simulink model "transform_test"  (R2021b)
settings: Solver=VariableStepAuto  StartTime=0.0  StopTime=60  RelTol=1e-3
libraries: simulink x1
settings Model: Creator=brian  LastModifiedBy=brian

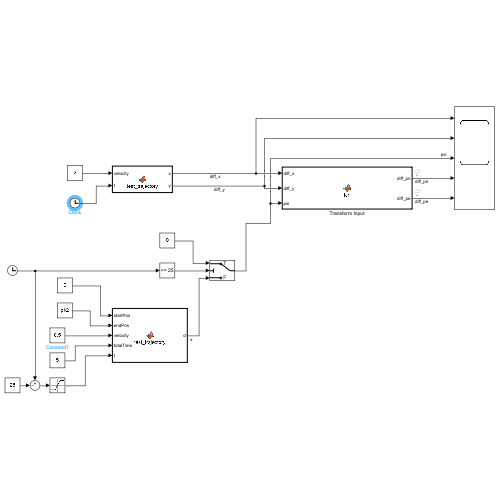
[thumbnail: Simulink's stored preview of the top-level diagram]
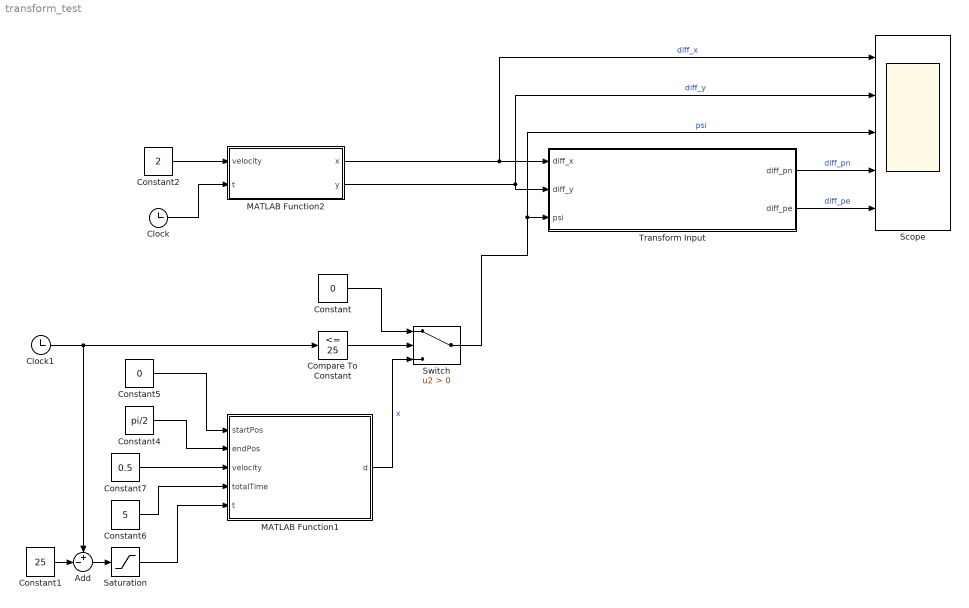
== system transform_test ==
  Add : Sum  Inputs=+-|
  Clock : Clock
  Clock1 : Clock
  Compare To Constant : simulink/Logic and Bit Operations/Compare To Constant  relop=<=  const=25  OutDataTypeStr=boolean
  Constant : Constant  Value=0
  Constant1 : Constant  Value=25
  Constant2 : Constant  Value=2
  Constant4 : Constant  Value=pi/2
  Constant5 : Constant  Value=0
  Constant6 : Constant  Value=5
  Constant7 : Constant  Value=0.5
  MATLAB Function1 : MATLAB Function  TreatAsAtomicUnit=on  SystemSampleTime=0.001
  MATLAB Function2 : MATLAB Function  TreatAsAtomicUnit=on  SystemSampleTime=0.001
  Saturation : Saturate  UpperLimit=250  LowerLimit=0
  Scope : Scope  NumInputPorts=5
  Switch : Switch  Criteria=u2 > Threshold
  Transform Input : MATLAB Function  TreatAsAtomicUnit=on
  wires:
  Transform Input/2(diff_pe) -> Scope/5  "diff_pe"
  Transform Input/1(diff_pn) -> Scope/4  "diff_pn"
  MATLAB Function2/2(y) -> Transform Input/2(diff_y), Scope/2  "diff_y"
  MATLAB Function2/1(x) -> Scope/1, Transform Input/1(diff_x)  "diff_x"
  Switch/1 -> Scope/3, Transform Input/3(psi)  "psi"
  Constant2/1 -> MATLAB Function2/1(velocity)
  Clock/1 -> MATLAB Function2/2(t)
  Constant1/1 -> Add/2
  Compare To Constant/1 -> Switch/2
  Saturation/1 -> MATLAB Function1/5(t)
  Add/1 -> Saturation/1
  Constant5/1 -> MATLAB Function1/1(startPos)
  Constant7/1 -> MATLAB Function1/3(velocity)
  MATLAB Function1/1(d) -> Switch/3  "x"
  Constant6/1 -> MATLAB Function1/4(totalTime)
  Constant/1 -> Switch/1
  Constant4/1 -> MATLAB Function1/2(endPos)
  Clock1/1 -> Compare To Constant/1, Add/1

== matlab function transform_test/MATLAB Function2 ==
  settings: updateMethod=DISCRETE
  data: velocity input; x output; t input; y output

function [x, y] = test_trajectory(velocity, t)
    x = LSPB(0, 72, t, velocity*2, 20);
    y = 0;
end

% function [x, y] = test_trajectory(velocity, t)
%     x = LSPB(0, 72, t, velocity*2, 20);
%     if (t < 22.5)
%         y = 0;
%     else
%         yt = t - 22.5;
%         y = LSPB(0, 110, yt, velocity*2, 30);
%     end
% end

== matlab function transform_test/MATLAB Function1 ==
  settings: updateMethod=DISCRETE
  data: startPos input; endPos input; velocity input; totalTime input; d output; t input
function d = test_trajectory(startPos, endPos, velocity, totalTime, t)
d = LSPB(startPos, endPos, t, velocity, totalTime);
end

== matlab function transform_test/Transform Input ==
  data: diff_x input; diff_pn output; diff_y input; psi input; diff_pe output
function [ diff_pn,  diff_pe] = fcn(diff_x, diff_y, psi)

diff_pn = diff_x*sin(pi/2 - psi) + diff_y*cos(pi/2 - psi);
diff_pe = -diff_x*cos(pi/2 - psi) + diff_y*sin(pi/2 - psi);

end
